simulink model "BHclientV"  (Simulink 7.4)
settings: Solver=ode3  StartTime=0.0  StopTime=inf  FixedStep=0.005  RelTol=1e-3
libraries: simulink_extras x1, planmant x1
settings Model: Creator=Admin  LastModifiedBy=Admin

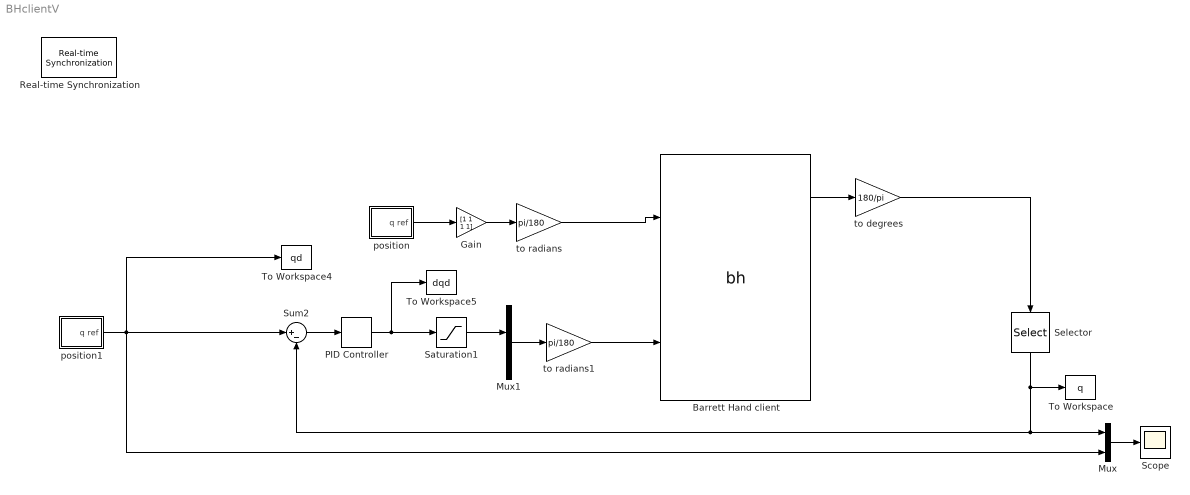
== system BHclientV ==
  Barrett Hand client : S-Function  FunctionName=bh  Parameters=IP port mode262 mode280 ST a0 a1 a2 a3 a4 a41 a5 a6 a7 a8 a81 a9  EnableBusSupport=off  mask(Barrett Hand UDP client){mode262=Velocity, mode280=Velocity, IP=193.2.6.168, port=4444, ST=0.005, a0=off, a1=off, a2=off, a3=off, a4=off, a41=off, a5=on, a6=on, a7=off, a8=off, a81=on, a9=off}
      mask prompts: mode262 "BH262 mode"; mode280 "BH280 mode"; port "UDP port"; a0 "Time"; a1 "262 position"; a2 "262 velocity"; a3 "262 deltap"; a4 "262 strain"; a41 "262 strain filt"; a5 "280 position"; a6 "280 velocity"; a7 "280 deltap"; a8 "280 strain"; a81 "280 strain filt"; a9 "pps"
      mask help:
      | Make sure you select the right mode. Sending positions when velocity mode
      | selected may not end well.
      |
      | Units are rad and rad/s. Strain and pps data is raw (no units)
      mask StyleString: popup(Velocity|Position|Torque|Other),popup(Velocity|Position|Torque|Other),edit,edit,edit,checkbox,checkbox,checkbox,checkbox,checkbox,checkbox,checkbox,checkbox,checkbox,checkbox,checkbox,checkbox
      mask CallbackString: togglePorts()|togglePorts()|togglePorts()|togglePorts()||togglePorts()|togglePorts()|togglePorts()|togglePorts()|togglePorts()|togglePorts()|togglePorts()|togglePorts()|togglePorts()|togglePorts()|togglePorts()|togglePorts()
      mask TabNameString: Control,Control,Control,Control,Control,Outputs,Outputs,Outputs,Outputs,Outputs,Outputs,Outputs,Outputs,Outputs,Outputs,Outputs,Outputs
      mask Display: text(0.3, 0.9, '\fontsize{10}IP: {\bf193.2.6.168 \newline\rmport: \bf4444}', 'horizontalAlignment', 'center','texmode','on')color('red')port_label('input',1,'\fontsize{12}BH262 {\newline\bfVelocity}','texmode','on')color('red') port_label('input',2,'\fontsize{12}BH280  {\newline\bfVelocity}','texmode','on')color('black')port_label('output',1,'\fontsize{11}BH280 {\bfPosition}','texmode','on');port_label('output',2,'BH280 {Velocity}','texmode','on');port_label('output',3,'BH280 {StrainFltr}','texmode','on');
  Gain : Gain  Gain=[1 1 1 1]  ParameterDataType=fixdt(1, 16)  ParameterScaling=2^0  OutDataType=fixdt(1, 16)  OutScaling=2^0
  Mux : Mux  Inputs=2
  Mux1 : Mux
  PID Controller : simulink_extras/Additional Linear/PID Controller  SystemSampleTime=-1  P=0.006  I=0  D=0
  Real-time Synchronization : planmant/Utility/Real-time Synchronization  SystemSampleTime=-1
  Saturation1 : Saturate  UpperLimit=0.1  LowerLimit=-0.1  OutDataType=fixdt(1, 16)  OutScaling=2^0
  Scope : Scope
      settings: TimeRange=10  YMin=30  YMax=100
  Selector : Selector  InputPortWidth=4  IndexOptions=Index vector (dialog)  Indices=2  OutputSizes=1
  Sum2 : Sum  Inputs=|+-  OutDataType=fixdt(1, 16)  OutScaling=2^0
  To Workspace : ToWorkspace  VariableName=q  SampleTime=-1  SaveFormat=Structure
  To Workspace4 : ToWorkspace  VariableName=qd  SampleTime=-1  SaveFormat=Structure With Time
  To Workspace5 : ToWorkspace  VariableName=dqd  SampleTime=-1  SaveFormat=Structure
  position : Subsystem
  position1 : Subsystem
  to degrees : Gain  Gain=180/pi  ParameterDataType=fixdt(1, 16)  ParameterScaling=2^0  OutDataType=fixdt(1, 16)  OutScaling=2^0
  to radians : Gain  Gain=pi/180  ParameterDataType=fixdt(1, 16)  ParameterScaling=2^0  OutDataType=fixdt(1, 16)  OutScaling=2^0
  to radians1 : Gain  Gain=pi/180  ParameterDataType=fixdt(1, 16)  ParameterScaling=2^0  OutDataType=fixdt(1, 16)  OutScaling=2^0
  wires:
  Selector/1 -> To Workspace/1, Mux/1, Sum2/2
  Gain/1 -> to radians/1
  position/1(q ref) -> Gain/1
  Mux1/1 -> to radians1/1
  to degrees/1 -> Selector/1
  position1/1(q ref) -> To Workspace4/1, Mux/2, Sum2/1
  to radians/1 -> Barrett Hand client/1
  PID Controller/1 -> To Workspace5/1, Saturation1/1
  Sum2/1 -> PID Controller/1
  to radians1/1 -> Barrett Hand client/2
  Mux/1 -> Scope/1
  Barrett Hand client/1 -> to degrees/1
  Saturation1/1 -> Mux1/2

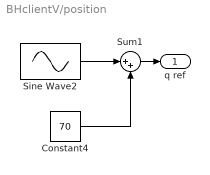
== system BHclientV/position ==
  Constant4 : Constant  Value=70  OutDataType=fixdt(1, 16)  OutScaling=2^0
  Sine Wave2 : Sin  Amplitude=30  Bias=0  Frequency=pi  Phase=pi/4  Samples=10  Offset=0
  Sum1 : Sum  Inputs=|++  OutDataType=fixdt(1, 16)  OutScaling=2^0
  q ref : Outport
  wires:
  Sum1/1 -> q ref/1
  Constant4/1 -> Sum1/2
  Sine Wave2/1 -> Sum1/1

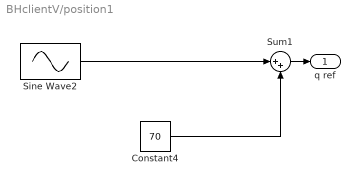
== system BHclientV/position1 ==
  Constant4 : Constant  Value=70  OutDataType=fixdt(1, 16)  OutScaling=2^0
  Sine Wave2 : Sin  Amplitude=30  Bias=0  Frequency=0.5*pi  Phase=pi/4  Samples=10  Offset=0
  Sum1 : Sum  Inputs=|++  OutDataType=fixdt(1, 16)  OutScaling=2^0
  q ref : Outport
  wires:
  Sum1/1 -> q ref/1
  Constant4/1 -> Sum1/2
  Sine Wave2/1 -> Sum1/1
